simulink model "nonlinearpendulum"  (R2018b)
settings: Solver=VariableStepAuto  StartTime=0.0  StopTime=5  RelTol=1e-3
values from neighbouring files (symbols this model uses):
  ctrl = lqr(A,B,Q,R)    [Pendulum.m]    (also in init_cranedamping_lqr.m)
  g = 9.82    [Pendulum.m]    (also in init_cranedamping.m; init_cranedamping_lqr.m)
  l = 0.3    [Pendulum.m]    (also in init_cranedamping.m; init_cranedamping_lqr.m)
  ref = 0    [Pendulum.m]    (also in init_cranedamping_lqr.m)
  theta_0 = pi/2    (= 1.57079632679)    [Pendulum.m]    (also in init_cranedamping_lqr.m)
settings Model: Creator=ola  LastModifiedBy=ola

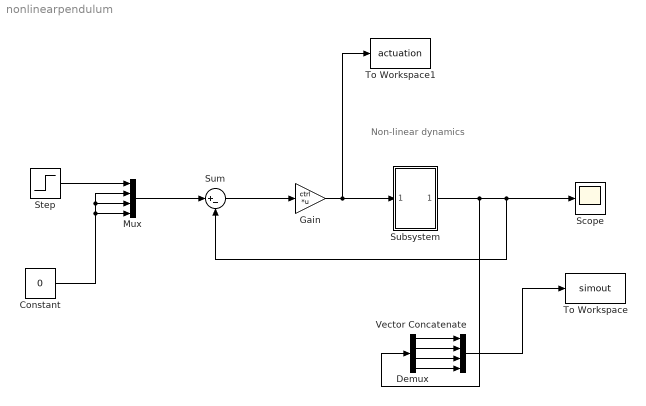
== system nonlinearpendulum ==
  note: Non-linear dynamics
  Constant : Constant  Value=0
  Demux : Demux
  Gain : Gain  Gain=ctrl  Multiplication=Matrix(K*u) (u vector)
  Mux : Mux
  Scope : Scope
  Step : Step  After=ref  SampleTime=0
  Subsystem : Subsystem
  Sum : Sum  Inputs=|+-
  To Workspace : ToWorkspace  VariableName=simout  SaveFormat=Timeseries  SampleTime=-1
  To Workspace1 : ToWorkspace  VariableName=actuation  SaveFormat=Timeseries  SampleTime=-1
  Vector Concatenate : Concatenate  NumInputs=4
  wires:
  Subsystem/1(Out1) -> Demux/1, Sum/2, Scope/1
  Gain/1 -> To Workspace1/1, Subsystem/1(In1)
  Sum/1 -> Gain/1
  Mux/1 -> Sum/1
  Step/1 -> Mux/1
  Constant/1 -> Mux/4, Mux/3, Mux/2
  Demux/1 -> Vector Concatenate/1
  Demux/2 -> Vector Concatenate/2
  Demux/3 -> Vector Concatenate/3
  Demux/4 -> Vector Concatenate/4
  Vector Concatenate/1 -> To Workspace/1

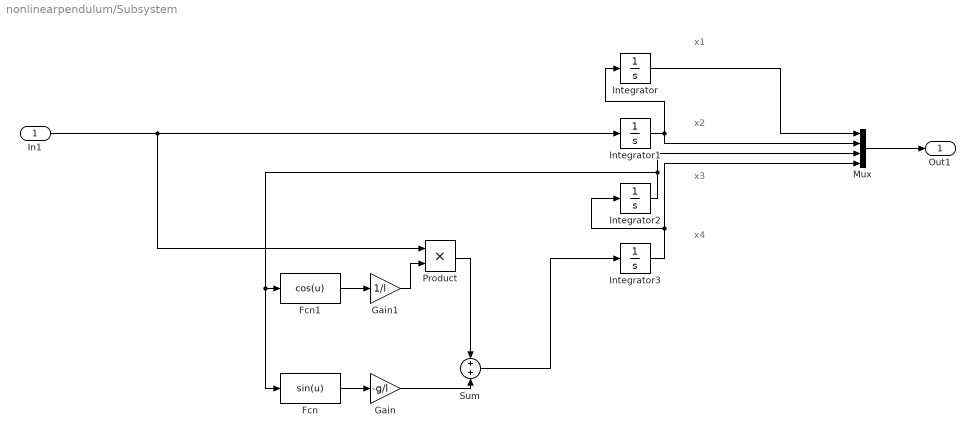
== system nonlinearpendulum/Subsystem ==
  note: x4
  note: x2
  note: x1
  note: x3
  In1 : Inport
  Fcn : Fcn  Expr=sin(u)
  Fcn1 : Fcn  Expr=cos(u)
  Gain : Gain  Gain=-g/l
  Gain1 : Gain  Gain=1/l
  Integrator : Integrator
  Integrator1 : Integrator
  Integrator2 : Integrator  InitialCondition=theta_0
  Integrator3 : Integrator
  Mux : Mux
  Product : Product
  Sum : Sum  Inputs=+|+
  Out1 : Outport
  wires:
  Gain1/1 -> Product/2
  Integrator3/1 -> Mux/4, Integrator2/1
  Integrator1/1 -> Mux/2, Integrator/1
  Product/1 -> Sum/1
  Gain/1 -> Sum/2
  Sum/1 -> Integrator3/1
  Fcn1/1 -> Gain1/1
  In1/1 -> Product/1, Integrator1/1
  Integrator2/1 -> Mux/3, Fcn1/1, Fcn/1
  Fcn/1 -> Gain/1
  Integrator/1 -> Mux/1
  Mux/1 -> Out1/1
